simulink model "adc_sim"  (R2015a)
settings: Solver=ode45  StartTime=5  StopTime=6  RelTol=1e-3
settings Model: Creator=henry  LastModifiedBy=henry

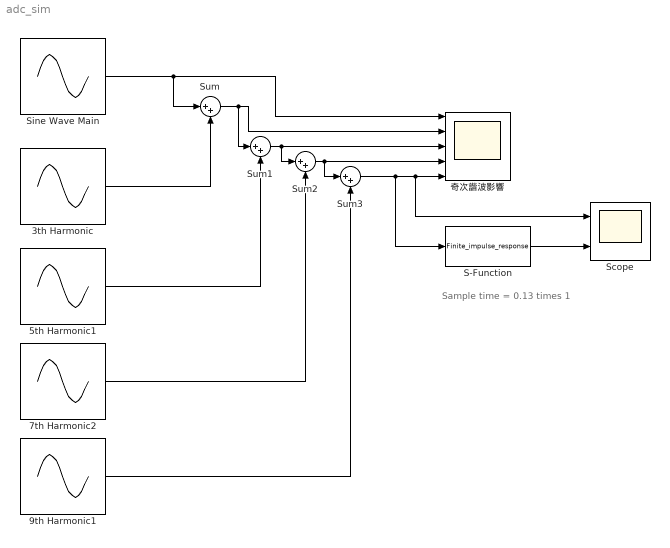
== system adc_sim ==
  note: Sample time = 0.13
      | times 1
  3th Harmonic : Sin  Amplitude=110  Frequency=377*3  SampleTime=0
  5th Harmonic1 : Sin  Amplitude=110  Frequency=377*5  SampleTime=0
  7th Harmonic2 : Sin  Amplitude=110  Frequency=377*7  SampleTime=0
  9th Harmonic1 : Sin  Amplitude=110  Frequency=377*9  SampleTime=0
  S-Function : S-Function  FunctionName=Finite_impulse_response  Parameters=0.13,1
  Scope : Scope  NumInputPorts=2
      settings: YMin=-5~-5  YMax=5~5  ScrollMode=on
  Sine Wave Main : Sin  Amplitude=110  Frequency=377  SampleTime=0
  Sum{,1..3} (4 alike) : Sum  Inputs=|++
  奇次諧波影響 : Scope  NumInputPorts=5
      settings: YMin=-5~-5~-5~-5~-5  YMax=5~5~5~5~5
  wires:
  Sine Wave Main/1 -> Sum/1, 奇次諧波影響/1
  3th Harmonic/1 -> Sum/2
  Sum/1 -> Sum1/1, 奇次諧波影響/2
  5th Harmonic1/1 -> Sum1/2
  Sum1/1 -> Sum2/1, 奇次諧波影響/3
  7th Harmonic2/1 -> Sum2/2
  Sum2/1 -> Sum3/1, 奇次諧波影響/4
  Sum3/1 -> S-Function/1, Scope/1, 奇次諧波影響/5
  9th Harmonic1/1 -> Sum3/2
  S-Function/1 -> Scope/2
